simulink model "P6"  (R2022b)
settings: Solver=VariableStepAuto  StartTime=0.0  StopTime=10.0  RelTol=1e-3
settings Model: Creator=andre  LastModifiedBy=andre

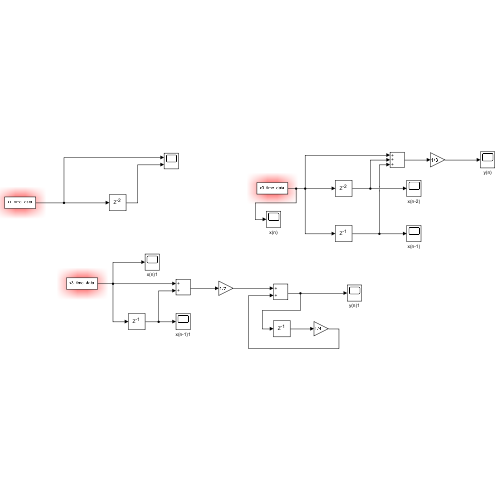
[thumbnail: Simulink's stored preview of the top-level diagram]
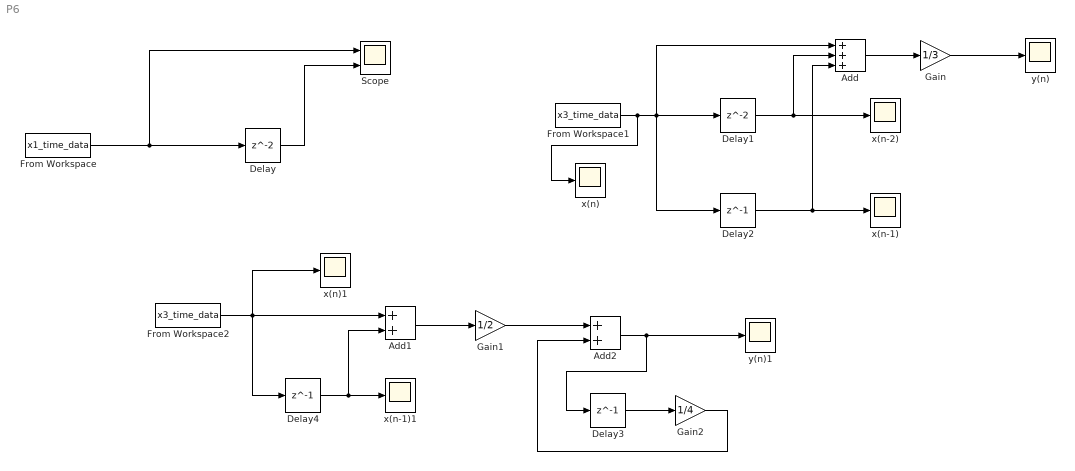
== system P6 ==
  Add : Sum  Inputs=+++
  Add1 : Sum
  Add2 : Sum
  Delay : Delay  InitialCondition=0
  Delay1 : Delay  InitialCondition=0
  Delay2 : Delay  DelayLength=1  InitialCondition=0
  Delay3 : Delay  DelayLength=1  InitialCondition=0
  Delay4 : Delay  DelayLength=1  InitialCondition=0
  From Workspace : FromWorkspace  VariableName=x1_time_data
  From Workspace1 : FromWorkspace  VariableName=x3_time_data
  From Workspace2 : FromWorkspace  VariableName=x3_time_data
  Gain : Gain  Gain=1/3
  Gain1 : Gain  Gain=1/2
  Gain2 : Gain  Gain=1/4
  Scope : Scope  NumInputPorts=2
  x(n) : Scope
  x(n)1 : Scope
  x(n-1) : Scope
  x(n-1)1 : Scope
  x(n-2) : Scope
  y(n) : Scope
  y(n)1 : Scope
  wires:
  From Workspace/1 -> Scope/1, Delay/1
  Delay/1 -> Scope/2
  Delay1/1 -> x(n-2)/1, Add/2
  Gain/1 -> y(n)/1
  From Workspace1/1 -> x(n)/1, Delay2/1, Add/1, Delay1/1
  Delay2/1 -> x(n-1)/1, Add/3
  Add/1 -> Gain/1
  Gain1/1 -> Add2/1
  Gain2/1 -> Add2/2
  Delay3/1 -> Gain2/1
  Add2/1 -> Delay3/1, y(n)1/1
  Add1/1 -> Gain1/1
  Delay4/1 -> Add1/2, x(n-1)1/1
  From Workspace2/1 -> x(n)1/1, Delay4/1, Add1/1
